simulink model "suspension"  (R2019a)
settings: Solver=ode15s  StartTime=0.0  StopTime=60  MaxStep=0.01  RelTol=1e-3  EnableMultiTasking=on
model workspace (MATLAB code in the model file):
  | dgrey = [0.3 0.3 0.3];
  | lgrey = [0.6 0.6 0.6];
  | orange = [255 140 0]/255;
  | blue = [0.0 0.6 0.8];
  | brown = [0.3 0.2 0.0];
  | lbrown = [167 108 52]/255;
  | yellow = [0.9 0.7 0.2];
  | red = [1.0 0.2 0.2];
  | black = [0 0 0];
  | 
  | rho_alum = 2700;
values from neighbouring files (symbols this model uses):
  back_frame_rad = intocm(0.25)    [loading.m]
  back_frame_thick_frame = intocm(0.25)    [loading.m]
  brake_disk_rad = intocm(3)    [loading.m]
  brake_disk_thick = intocm(0.25)    [loading.m]
  front_frame_rad = intocm(0.25)    [loading.m]
  front_frame_thick_frame = intocm(0.25)    [loading.m]
  hub_radius = intocm(2)    [loading.m]
  lower_left_link_len = intocm(link_upper)    [loading.m]
  lower_right_link_len = intocm(link_upper)    [loading.m]
  max_angle = 35    [loading.m]
  num_spokes = 4    [loading.m]
  outer_radius_spokes = intocm(5)    [loading.m]
  shaft_len = intocm(8)    [loading.m]
  shaft_rad = intocm(1.5)    [loading.m]
  steer_arm_chamfer = 0.25    [loading.m]
  steer_arm_height_forked = 13    [loading.m]
  steer_arm_len = 20    [loading.m]
  steer_arm_len_forked = 4    [loading.m]
  steer_arm_offset_forked = 3    [loading.m]
  steer_arm_pin_rad = 0.25    [loading.m]
  steer_arm_thick = 1    [loading.m]
  steer_arm_width = 2    [loading.m]
  steering_ball_rad = 1    [loading.m]
  steering_pin_height = 3    [loading.m]
  steering_pin_rad = 0.5    [loading.m]
  thickness_spokes = intocm(1)    [loading.m]
  tire_chamfer = 1    [loading.m]
  tire_density = 1000    [loading.m]
  tire_radius = intocm(9)    [loading.m]
  tire_width = intocm(7.5)    [loading.m]
  Ts = 60    [loading.m]
  upper_left_link_len = intocm(link_upper)    [loading.m]
  upper_right_link_len = intocm(link_upper)    [loading.m]
  upright_bearing_housing = 6    [loading.m]
  upright_chamfer = 0.3    [loading.m]
  upright_heigh_wheel = 8    [loading.m]
  upright_height = 43    [loading.m]
  upright_hub_thick = 2.5    [loading.m]
  upright_len = 8    [loading.m]
  upright_shaft_rad = 2.5    [loading.m]
  upright_thickness = 1    [loading.m]
  upright_trans_rad_to_wheel = 2    [loading.m]
  upright_width_wishbone = 10    [loading.m]
  width_hub = intocm(4.5)    [loading.m]
undefined symbols (not defined in the file or in its folder): sm_dwb_roadgen, X, Y, Z
libraries: sm_lib x75, sm_double_wishbone_suspension_lib x23, nesl_utility x18, simulink x3
(part 2 of 4)

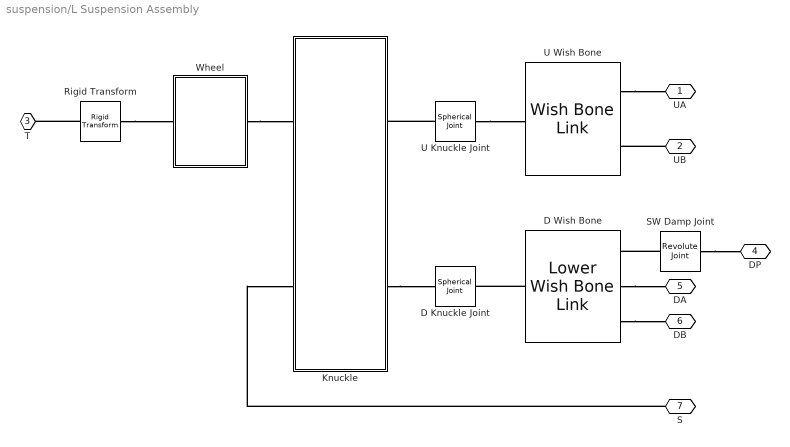
== system suspension/L Suspension Assembly ==
  D Knuckle Joint : sm_lib/Joints/Spherical Joint  SenseConstraintForce=off  SenseConstraintForceX=off  SenseConstraintForceY=off  SenseConstraintForceZ=off  SenseConstraintTorque=off  SenseConstraintTorqueX=off  SenseConstraintTorqueY=off  SenseConstraintTorqueZ=off  SenseTotalForce=off  SenseTotalForceX=off  SenseTotalForceY=off  SenseTotalForceZ=off  SenseTotalTorque=off  SenseTotalTorqueX=off  SenseTotalTorqueY=off  SenseTotalTorqueZ=off  CompositeWrenchDir=FollowerOnBase  CompositeWrenchFrame=BaseFrame  DefPosRotationMethod=None  DefPosRotationAngleUnits=deg  DefPosRotationStandardAxis=+Z  DefPosRotationAngle=0  DefPosRotationArbitraryAxis=[0 0 1]  DefPosFollAlignAxisA=+X  DefPosBaseAlignAxisA=+Y  DefPosFollAlignAxisB=+Y  DefPosBaseAlignAxisB=+Z  DefPosRotationSequenceAxes=FollowerAxes  DefPosRotationSequence=XYX  DefPosRotationSequenceAngles=[0 0 0]  DefPosRotationSequenceAnglesUnits=deg  DefPosRotationMatrix=[1 0 0; 0 1 0; 0 0 1]  EqPosRotationMethod=None  EqPosRotationAngleUnits=deg  EqPosRotationStandardAxis=+Z  EqPosRotationAngle=0  EqPosRotationArbitraryAxis=[0 0 1]  EqPosFollAlignAxisA=+X  EqPosBaseAlignAxisA=+Y  EqPosFollAlignAxisB=+Y  EqPosBaseAlignAxisB=+Z  EqPosRotationSequenceAxes=FollowerAxes  EqPosRotationSequence=XYX  EqPosRotationSequenceAngles=[0 0 0]  EqPosRotationSequenceAnglesUnits=deg  EqPosRotationMatrix=[1 0 0; 0 1 0; 0 0 1]  SpringStiffness=0  SpringStiffnessUnits=N*m/deg  DampingCoefficient=0  DampingCoefficientUnits=N*m/(deg/s)  ActuateTorqueX=off  ActuateTorqueY=off  ActuateTorqueZ=off  ActuateTorque=off  TorqueActuationMode=NoTorque  MotionActuationMode=ComputedMotion  ActuationFrame=BaseFrame  SensePosition=off  SenseVelocityX=off  SenseVelocityY=off  SenseVelocityZ=off  SenseVelocity=off  SenseAccelerationX=off  SenseAccelerationY=off  SenseAccelerationZ=off  SenseAcceleration=off  SenseTorqueX=off  SenseTorqueY=off  SenseTorqueZ=off  SenseTorqueForce=off  SenseLowerLimitTorqueMag=off  SenseUpperLimitTorqueMag=off  SensingFrame=BaseFrame  LowerLimitSpecify=off  LowerLimitBound=15  LowerLimitBoundUnits=deg  LowerLimitStiffness=1e4  LowerLimitStiffnessUnits=N*m/deg  LowerLimitDamping=10  LowerLimitDampingUnits=N*m/(deg/s)  LowerLimitTransitionRegionWidth=0.1  LowerLimitTransitionRegionWidthUnits=deg  UpperLimitSpecify=off  UpperLimitBound=45  UpperLimitBoundUnits=deg  UpperLimitStiffness=1e4  UpperLimitStiffnessUnits=N*m/deg  UpperLimitDamping=10  UpperLimitDampingUnits=N*m/(deg/s)  UpperLimitTransitionRegionWidth=0.1  UpperLimitTransitionRegionWidthUnits=deg  PositionTargetRotationMethod=None  PositionTargetRotationAngleUnits=deg  PositionTargetRotationStandardAxis=+Z  PositionTargetRotationAngle=0  PositionTargetRotationArbitraryAxis=[0 0 1]  PositionTargetFollAlignAxisA=+Y  PositionTargetBaseAlignAxisA=-Y  PositionTargetFollAlignAxisB=+Z  PositionTargetBaseAlignAxisB=-Z  PositionTargetRotationSequenceAxes=FollowerAxes  PositionTargetRotationSequence=XYX  PositionTargetRotationSequenceAngles=[0 0 0]  PositionTargetRotationSequenceAnglesUnits=deg  PositionTargetRotationMatrix=[1 0 0; 0 1 0; 0 0 1]  PositionTargetSpecify=off  PositionTargetPriority=Low  VelocityTargetValue=[0 0 0]  VelocityTargetValueUnits=deg/s  VelocityTargetSpecify=off  VelocityTargetPriority=High  VelocityTargetInFollowerFrame=on
  D Wish Bone : sm_double_wishbone_suspension_lib/Lower Wish Bone Link  L1=36  L2=25  L3=5  W3=5  W=14.75  T=2  Rb=2.875  Ob=15  Rev=on  Lb=4  Rsh=0.75  Rs=2  Hi=1.4  Rh=1  Oh=3.0625  Odb=10  Wdb=4  Ldb=4  Tdb=1  Sdb=1.5  Rhdb=1  rho=rho_alum  clr=lbrown
      settings: SourceProductName=Simscape Multibody  SourceProductBaseCode=MS
  Knuckle : Subsystem  mask(Steering knuckle){H=upright_height, L=upright_len, T=upright_thickness, Wpr=upright_hub_thick, Hpr=upright_heigh_wheel, Wc=upright_width_wishbone, Rd=upright_shaft_rad, Hd=upright_bearing_housing, Rr=upright_chamfer, Rt=upright_trans_rad_to_wheel, Rb=steering_ball_rad, Rp=steering_pin_rad, Hp=steering_pin_height, Ls=steer_arm_len, Ws=steer_arm_width, Ts=steer_arm_thick, Hsf=steer_arm_height_forked, Lsf=steer_arm_len_forked, Osf=steer_arm_offset_forked, Rsp=steer_arm_pin_rad, Rsr=steer_arm_chamfer, Rev=on, rho=rho_alum, clr=dgrey}
      mask prompts: H "Height (cm):"; L "Length (cm):"; T "Thickness (cm):"; Wpr "Width of wheel attach projection (cm):"; Hpr "Height of wheel attach projection (cm):"; Wc "Width of wishbone connectors (cm):"; Rd "Drive shaft hole radius (cm):"; Hd "Drive shaft bearing housing height (cm):"; Rr "Chamfer/fillet radius (cm):"; Rt "Transition radius to wheel attach projection (cm):"; Rb "Ball radius (cm):"; Rp "Pin radius (cm):"; Hp "Pin height (cm):"; Ls "Length of arm (cm):"; Ws "Width of arm (cm):"; Ts "Thickness of arm (cm):"; Hsf "Height of forked section (cm):"; Lsf "Length of forked section (cm):"; Osf "Offset of forked section (cm):"; Rsp "Pin radius (cm):"; Rsr "Chamfer/fillet radius (cm):"; Rev "Reverse direction:"; rho "Density (kg/m^3):"; clr "Color [r g b]:"
      mask help: This block models a steering knuckle. The wheel hub attaches to the steering knuckle. The steering knuckle attaches to the wishbone links. The ports U and D correspond to the frames where the knucle connects to the wishbone links. The port W corresponds to the frame where the wheel hub attaches to the knuckle. The knuckle also has a rigidly attached steering arm that attaches to the steering rack via tie rods. The port S corresponds to the frame where the steering arm attaches to the tie rod.
      mask init:
      | s_knuckle_xsec = [0 -Hd/2; 0 -Hpr/2; Wpr -Hpr/2; Wpr -H/2;
      |                 Wpr+Wc -H/2; Wpr+Wc -H/2+T; Wpr+T -H/2+T;
      |                  Wpr+T -Hd/2];
      | 
      | s_knuckle_xsec = simmechanics.demohelpers.round_corners(s_knuckle_xsec, 2:7, ...
      |                              [Rr Rt Rr*ones(1,4)], 20);
      | 
      | n_knuckle_xsec = flipud([s_knuckle_xsec(:,1) -s_knuckle_xsec(:,2)]);                         
      | 
      | Roh = sqrt((L/2)^2 + (Hd/2)^2);
      | phi = atan2(Hd,L);
      | theta = linspace(pi/2-phi,pi/2+phi,50)';
      | sh_xsec = [Roh*cos(theta) Roh*sin(theta)];
      | theta = linspace(3*pi/2-phi,3*pi/2+phi,50)';
      | sh_xsec = [sh_xsec; Roh*cos(theta) Roh*sin(theta)];
      | theta = linspace(5*pi/2-phi,pi/2-phi,100)';
      | sh_xsec = [sh_xsec; sh_xsec(1,:); Rd*cos(theta) Rd*sin(theta)];
      | 
      | % Convert Rev variable into +/- 1 instead of 0 or 1
      | sgn = (2*Rev-1);
      mask Display:
      | image(imread('sm_dwishbone_knuckle.png'));
      | port_label('RConn',1,'U');
      | port_label('RConn',2,'D');
      | port_label('LConn',1,'W');
      | port_label('LConn',2,'S');
  Rigid Transform : sm_lib/Frames and Transforms/Rigid Transform  TranslationMethod=None  TranslationStandardOffset=0  TranslationLengthUnit=m  TranslationStandardAxis=+Z  TranslationCartesianOffset=[0 0 0]  TranslationROffset=0  TranslationROffsetUnits=m  TranslationZOffset=0  TranslationZOffsetUnits=m  TranslationThetaOffset=0  TranslationThetaOffsetUnits=deg  RotationMethod=AlignedAxes  RotationAngleUnits=deg  RotationStandardAxis=+Z  RotationAngle=0  RotationArbitraryAxis=[0 0 1]  FollAlignAxisA=+X  BaseAlignAxisA=-X  FollAlignAxisB=+Z  BaseAlignAxisB=+Z  RotationSequenceAxes=FollowerAxes  RotationSequence=XYX  RotationSequenceAngles=[0 0 0]  RotationSequenceAnglesUnits=deg  RotationMatrix=[1 0 0; 0 1 0; 0 0 1]
  SW Damp Joint : sm_lib/Joints/Revolute Joint  SenseConstraintForce=off  SenseConstraintForceX=off  SenseConstraintForceY=off  SenseConstraintForceZ=off  SenseConstraintTorque=off  SenseConstraintTorqueX=off  SenseConstraintTorqueY=off  SenseConstraintTorqueZ=off  SenseTotalForce=off  SenseTotalForceX=off  SenseTotalForceY=off  SenseTotalForceZ=off  SenseTotalTorque=off  SenseTotalTorqueX=off  SenseTotalTorqueY=off  SenseTotalTorqueZ=off  CompositeWrenchDir=FollowerOnBase  CompositeWrenchFrame=BaseFrame  EquilibriumPosition=0  EquilibriumPositionUnits=deg  SpringStiffness=0  SpringStiffnessUnits=N*m/deg  DampingCoefficient=0  DampingCoefficientUnits=N*m/(deg/s)  TorqueActuationMode=NoTorque  MotionActuationMode=ComputedMotion  SensePosition=off  SenseVelocity=off  SenseAcceleration=off  SenseTorqueForce=off  SenseLowerLimitTorqueForce=off  SenseUpperLimitTorqueForce=off  LowerLimitSpecify=off  LowerLimitBound=-90  LowerLimitBoundUnits=deg  LowerLimitStiffness=1e4  LowerLimitStiffnessUnits=N*m/deg  LowerLimitDamping=10  LowerLimitDampingUnits=N*m/(deg/s)  LowerLimitTransitionRegionWidth=0.1  LowerLimitTransitionRegionWidthUnits=deg  UpperLimitSpecify=off  UpperLimitBound=90  UpperLimitBoundUnits=deg  UpperLimitStiffness=1e4  UpperLimitStiffnessUnits=N*m/deg  UpperLimitDamping=10  UpperLimitDampingUnits=N*m/(deg/s)  UpperLimitTransitionRegionWidth=0.1  UpperLimitTransitionRegionWidthUnits=deg  PositionTargetSpecify=on  PositionTargetPriority=Low  PositionTargetValue=-30  PositionTargetValueUnits=deg  VelocityTargetSpecify=off  VelocityTargetPriority=High  VelocityTargetValue=0  VelocityTargetValueUnits=deg/s
  U Knuckle Joint : sm_lib/Joints/Spherical Joint  SenseConstraintForce=off  SenseConstraintForceX=off  SenseConstraintForceY=off  SenseConstraintForceZ=off  SenseConstraintTorque=off  SenseConstraintTorqueX=off  SenseConstraintTorqueY=off  SenseConstraintTorqueZ=off  SenseTotalForce=off  SenseTotalForceX=off  SenseTotalForceY=off  SenseTotalForceZ=off  SenseTotalTorque=off  SenseTotalTorqueX=off  SenseTotalTorqueY=off  SenseTotalTorqueZ=off  CompositeWrenchDir=FollowerOnBase  CompositeWrenchFrame=BaseFrame  DefPosRotationMethod=None  DefPosRotationAngleUnits=deg  DefPosRotationStandardAxis=+Z  DefPosRotationAngle=0  DefPosRotationArbitraryAxis=[0 0 1]  DefPosFollAlignAxisA=+X  DefPosBaseAlignAxisA=+Y  DefPosFollAlignAxisB=+Y  DefPosBaseAlignAxisB=+Z  DefPosRotationSequenceAxes=FollowerAxes  DefPosRotationSequence=XYX  DefPosRotationSequenceAngles=[0 0 0]  DefPosRotationSequenceAnglesUnits=deg  DefPosRotationMatrix=[1 0 0; 0 1 0; 0 0 1]  EqPosRotationMethod=None  EqPosRotationAngleUnits=deg  EqPosRotationStandardAxis=+Z  EqPosRotationAngle=0  EqPosRotationArbitraryAxis=[0 0 1]  EqPosFollAlignAxisA=+X  EqPosBaseAlignAxisA=+Y  EqPosFollAlignAxisB=+Y  EqPosBaseAlignAxisB=+Z  EqPosRotationSequenceAxes=FollowerAxes  EqPosRotationSequence=XYX  EqPosRotationSequenceAngles=[0 0 0]  EqPosRotationSequenceAnglesUnits=deg  EqPosRotationMatrix=[1 0 0; 0 1 0; 0 0 1]  SpringStiffness=0  SpringStiffnessUnits=N*m/deg  DampingCoefficient=0  DampingCoefficientUnits=N*m/(deg/s)  ActuateTorqueX=off  ActuateTorqueY=off  ActuateTorqueZ=off  ActuateTorque=off  TorqueActuationMode=NoTorque  MotionActuationMode=ComputedMotion  ActuationFrame=BaseFrame  SensePosition=off  SenseVelocityX=off  SenseVelocityY=off  SenseVelocityZ=off  SenseVelocity=off  SenseAccelerationX=off  SenseAccelerationY=off  SenseAccelerationZ=off  SenseAcceleration=off  SenseTorqueX=off  SenseTorqueY=off  SenseTorqueZ=off  SenseTorqueForce=off  SenseLowerLimitTorqueMag=off  SenseUpperLimitTorqueMag=off  SensingFrame=BaseFrame  LowerLimitSpecify=off  LowerLimitBound=15  LowerLimitBoundUnits=deg  LowerLimitStiffness=1e4  LowerLimitStiffnessUnits=N*m/deg  LowerLimitDamping=10  LowerLimitDampingUnits=N*m/(deg/s)  LowerLimitTransitionRegionWidth=0.1  LowerLimitTransitionRegionWidthUnits=deg  UpperLimitSpecify=off  UpperLimitBound=45  UpperLimitBoundUnits=deg  UpperLimitStiffness=1e4  UpperLimitStiffnessUnits=N*m/deg  UpperLimitDamping=10  UpperLimitDampingUnits=N*m/(deg/s)  UpperLimitTransitionRegionWidth=0.1  UpperLimitTransitionRegionWidthUnits=deg  PositionTargetRotationMethod=AlignedAxes  PositionTargetRotationAngleUnits=deg  PositionTargetRotationStandardAxis=+Z  PositionTargetRotationAngle=0  PositionTargetRotationArbitraryAxis=[0 0 1]  PositionTargetFollAlignAxisA=+X  PositionTargetBaseAlignAxisA=-X  PositionTargetFollAlignAxisB=+Z  PositionTargetBaseAlignAxisB=-Z  PositionTargetRotationSequenceAxes=FollowerAxes  PositionTargetRotationSequence=XYX  PositionTargetRotationSequenceAngles=[0 0 0]  PositionTargetRotationSequenceAnglesUnits=deg  PositionTargetRotationMatrix=[1 0 0; 0 1 0; 0 0 1]  PositionTargetSpecify=off  PositionTargetPriority=High  VelocityTargetValue=[0 0 0]  VelocityTargetValueUnits=deg/s  VelocityTargetSpecify=off  VelocityTargetPriority=High  VelocityTargetInFollowerFrame=on
  U Wish Bone : sm_double_wishbone_suspension_lib/Wish Bone Link  L1=25  L2=15  L3=5  W3=5  W=25  T=2  Rb=8  Ob=5  Rev=on  Lb=4  Rsh=0.75  Rs=2  Hi=1.4  Rh=1  Oh=3  rho=rho_alum  clr=brown
      settings: SourceProductName=Simscape Multibody  SourceProductBaseCode=MS
  Wheel : Subsystem  mask(Wheel){Rti=outer_radius_spokes, Rto=tire_radius, Wt=tire_width, Rtr=tire_chamfer, trho=tire_density, tclr=black, Rhi=hub_radius, Rho=outer_radius_spokes, Ns=num_spokes, Ts=thickness_spokes, Wh=width_hub, Ls=shaft_len, Rs=shaft_rad, Rb=brake_disk_rad, Tb=brake_disk_thick, srho=rho_alum, sclr=yellow}
      mask prompts: Rti "Tire inner radius (cm):"; Rto "Tire outer radius (cm):"; Wt "Tire width (cm):"; Rtr "Chamfer/fillet radius (cm):"; trho "Density (kg/m^3):"; tclr "Color [r  g b]:"; Rhi "Hub radius (cm):"; Rho "Outer radius of spokes (cm):"; Ns "Number of spokes:"; Ts "Thickness of spokes:"; Wh "Width of hub (cm):"; Ls "Shaft length (cm):"; Rs "Shaft radius (cm):"; Rb "Brake disc radius (cm):"; Tb "Brake disc thickness (cm):"; srho "Density (kg/m^3):"; sclr "Color [r g b]:"
      mask help: This block models a wheel assembly. The port H corresponds to the center of the wheel hub.
      mask init:
      | spk_angles = linspace(0,2*pi,Ns+1);
      | 
      | spokes_xsec = [];
      | r_indices = [];
      | wang = 20*pi/180;
      | for idx = 1:length(spk_angles)-1
      |     ang = spk_angles(idx);
      |     theta = linspace(ang-wang,ang+wang,20)';
      |     spokes_xsec = [spokes_xsec;
      |                    Rhi*cos(theta) Rhi*sin(theta)];
      |     theta = linspace(ang+wang, spk_angles(idx+1)-wang, 50)';
      |     len = length(spokes_xsec);
      |     r_indices = [r_indices len len+1];
      |     spokes_xsec = [spokes_xsec;
      |                    Rho*cos(theta) Rho*sin(theta)];
      | end
      | 
      | rim_xsec = [Rho -Wh/2; Rti -Wt/2; 
      |             Rti Wt/2; Rho Wh/2+Ts];
      | 
      | tire_xsec = [Rti -Wt/2; Rto -Wt/2; Rto Wt/2; Rti Wt/2];
      | tire_xsec = simmechanics.demohelpers.round_corners(tire_xsec,1:4,Rtr,10);
      mask Display:
      | image(imread('sm_dwishbone_wheel.png'));
      | port_label('LConn',1,'H');
      | port_label('RConn',1,'T');
  UA : PMIOPort  Side=Right
  UB : PMIOPort  Port=2  Side=Right
  T : PMIOPort  Port=3  Side=Left
  DP : PMIOPort  Port=4  Side=Right
  DA : PMIOPort  Port=5  Side=Right
  DB : PMIOPort  Port=6  Side=Right
  S : PMIOPort  Port=7  Side=Right
  connections:
  D Wish Bone/RConn1 -- D Knuckle Joint/LConn1
  Wheel/LConn1 -- Knuckle/LConn1
  D Wish Bone/LConn3 -- DB/RConn1
  D Wish Bone/LConn2 -- DA/RConn1
  U Wish Bone/LConn1 -- UA/RConn1
  UB/RConn1 -- U Wish Bone/LConn2
  U Knuckle Joint/RConn1 -- Knuckle/RConn1
  U Knuckle Joint/LConn1 -- U Wish Bone/RConn1
  Rigid Transform/LConn1 -- Wheel/RConn1
  Rigid Transform/RConn1 -- T/RConn1
  S/RConn1 -- Knuckle/LConn2
  Knuckle/RConn2 -- D Knuckle Joint/RConn1
  SW Damp Joint/LConn1 -- D Wish Bone/LConn1
  SW Damp Joint/RConn1 -- DP/RConn1

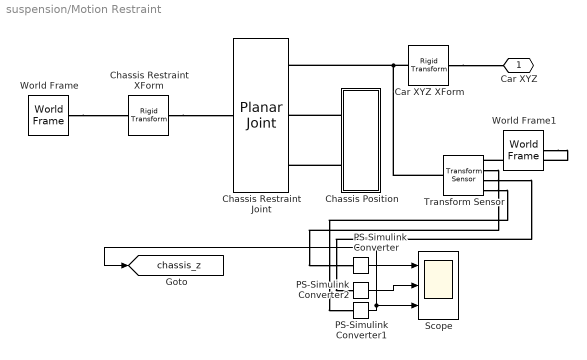
== system suspension/Motion Restraint ==
  Car XYZ XForm : sm_lib/Frames and Transforms/Rigid Transform  TranslationMethod=None  TranslationStandardOffset=0  TranslationLengthUnit=m  TranslationStandardAxis=+Z  TranslationCartesianOffset=[0 0 0]  TranslationROffset=0  TranslationROffsetUnits=m  TranslationZOffset=0  TranslationZOffsetUnits=m  TranslationThetaOffset=0  TranslationThetaOffsetUnits=deg  RotationMethod=AlignedAxes  RotationAngleUnits=deg  RotationStandardAxis=+Z  RotationAngle=0  RotationArbitraryAxis=[0 0 1]  FollAlignAxisA=+Y  BaseAlignAxisA=+X  FollAlignAxisB=+X  BaseAlignAxisB=+Z  RotationSequenceAxes=FollowerAxes  RotationSequence=XYX  RotationSequenceAngles=[0 0 0]  RotationSequenceAnglesUnits=deg  RotationMatrix=[1 0 0; 0 1 0; 0 0 1]
  Chassis Position : Subsystem
  Chassis Restraint XForm : sm_lib/Frames and Transforms/Rigid Transform  TranslationMethod=None  TranslationStandardOffset=0  TranslationLengthUnit=m  TranslationStandardAxis=+Z  TranslationCartesianOffset=[0 0 0]  TranslationROffset=0  TranslationROffsetUnits=m  TranslationZOffset=0  TranslationZOffsetUnits=m  TranslationThetaOffset=0  TranslationThetaOffsetUnits=deg  RotationMethod=AlignedAxes  RotationAngleUnits=deg  RotationStandardAxis=+Z  RotationAngle=0  RotationArbitraryAxis=[0 0 1]  FollAlignAxisA=+Y  BaseAlignAxisA=+Z  FollAlignAxisB=+X  BaseAlignAxisB=+X  RotationSequenceAxes=FollowerAxes  RotationSequence=XYX  RotationSequenceAngles=[0 0 0]  RotationSequenceAnglesUnits=deg  RotationMatrix=[1 0 0; 0 1 0; 0 0 1]
  Chassis Restraint Joint : sm_lib/Joints/Planar Joint  SenseConstraintForce=off  SenseConstraintForceX=off  SenseConstraintForceY=off  SenseConstraintForceZ=off  SenseConstraintTorque=off  SenseConstraintTorqueX=off  SenseConstraintTorqueY=off  SenseConstraintTorqueZ=off  SenseTotalForce=off  SenseTotalForceX=off  SenseTotalForceY=off  SenseTotalForceZ=off  SenseTotalTorque=off  SenseTotalTorqueX=off  SenseTotalTorqueY=off  SenseTotalTorqueZ=off  CompositeWrenchDir=FollowerOnBase  CompositeWrenchFrame=BaseFrame  PxEquilibriumPosition=0  PxEquilibriumPositionUnits=m  PxSpringStiffness=0  PxSpringStiffnessUnits=N/m  PxDampingCoefficient=0  PxDampingCoefficientUnits=N/(m/s)  PxTorqueActuationMode=NoTorque  PxMotionActuationMode=ComputedMotion  PxSensePosition=off  PxSenseVelocity=off  PxSenseAcceleration=off  PxSenseTorqueForce=off  PxSenseLowerLimitTorqueForce=off  PxSenseUpperLimitTorqueForce=off  PxLowerLimitSpecify=off  PxLowerLimitBound=-1  PxLowerLimitBoundUnits=m  PxLowerLimitStiffness=1e6  PxLowerLimitStiffnessUnits=N/m  PxLowerLimitDamping=1e3  PxLowerLimitDampingUnits=N/(m/s)  PxLowerLimitTransitionRegionWidth=1e-4  PxLowerLimitTransitionRegionWidthUnits=m  PxUpperLimitSpecify=off  PxUpperLimitBound=1  PxUpperLimitBoundUnits=m  PxUpperLimitStiffness=1e6  PxUpperLimitStiffnessUnits=N/m  PxUpperLimitDamping=1e3  PxUpperLimitDampingUnits=N/(m/s)  PxUpperLimitTransitionRegionWidth=1e-4  PxUpperLimitTransitionRegionWidthUnits=m  PxPositionTargetSpecify=off  PxPositionTargetPriority=High  PxPositionTargetValue=0  PxPositionTargetValueUnits=m  PxVelocityTargetSpecify=off  PxVelocityTargetPriority=High  PxVelocityTargetValue=0  PxVelocityTargetValueUnits=m/s  PyEquilibriumPosition=0  PyEquilibriumPositionUnits=m  PySpringStiffness=0  PySpringStiffnessUnits=N/m  PyDampingCoefficient=0  PyDampingCoefficientUnits=N/(m/s)  PyTorqueActuationMode=NoTorque  PyMotionActuationMode=ComputedMotion  PySensePosition=on  PySenseVelocity=off  PySenseAcceleration=off  PySenseTorqueForce=off  PySenseLowerLimitTorqueForce=off  PySenseUpperLimitTorqueForce=off  PyLowerLimitSpecify=off  PyLowerLimitBound=-1  PyLowerLimitBoundUnits=m  PyLowerLimitStiffness=1e6  PyLowerLimitStiffnessUnits=N/m  PyLowerLimitDamping=1e3  PyLowerLimitDampingUnits=N/(m/s)  PyLowerLimitTransitionRegionWidth=1e-4  PyLowerLimitTransitionRegionWidthUnits=m  PyUpperLimitSpecify=off  PyUpperLimitBound=1  PyUpperLimitBoundUnits=m  PyUpperLimitStiffness=1e6  PyUpperLimitStiffnessUnits=N/m  PyUpperLimitDamping=1e3  PyUpperLimitDampingUnits=N/(m/s)  PyUpperLimitTransitionRegionWidth=1e-4  PyUpperLimitTransitionRegionWidthUnits=m  PyPositionTargetSpecify=on  PyPositionTargetPriority=High  PyPositionTargetValue=95  PyPositionTargetValueUnits=cm  PyVelocityTargetSpecify=off  PyVelocityTargetPriority=High  PyVelocityTargetValue=0  PyVelocityTargetValueUnits=m/s  RzEquilibriumPosition=0  RzEquilibriumPositionUnits=deg  RzSpringStiffness=0  RzSpringStiffnessUnits=N*m/deg  RzDampingCoefficient=0  RzDampingCoefficientUnits=N*m/(deg/s)  RzTorqueActuationMode=NoTorque  RzMotionActuationMode=ComputedMotion  RzSensePosition=on  RzSenseVelocity=off  RzSenseAcceleration=off  RzSenseTorqueForce=off  RzSenseLowerLimitTorqueForce=off  RzSenseUpperLimitTorqueForce=off  RzLowerLimitSpecify=off  RzLowerLimitBound=-90  RzLowerLimitBoundUnits=deg  RzLowerLimitStiffness=1e4  RzLowerLimitStiffnessUnits=N*m/deg  RzLowerLimitDamping=10  RzLowerLimitDampingUnits=N*m/(deg/s)  RzLowerLimitTransitionRegionWidth=0.1  RzLowerLimitTransitionRegionWidthUnits=deg  RzUpperLimitSpecify=off  RzUpperLimitBound=90  RzUpperLimitBoundUnits=deg  RzUpperLimitStiffness=1e4  RzUpperLimitStiffnessUnits=N*m/deg  RzUpperLimitDamping=10  RzUpperLimitDampingUnits=N*m/(deg/s)  RzUpperLimitTransitionRegionWidth=0.1  RzUpperLimitTransitionRegionWidthUnits=deg  RzPositionTargetSpecify=on  RzPositionTargetPriority=High  RzPositionTargetValue=0  RzPositionTargetValueUnits=deg  RzVelocityTargetSpecify=off  RzVelocityTargetPriority=High  RzVelocityTargetValue=0  RzVelocityTargetValueUnits=deg/s
  PS-Simulink Converter : nesl_utility/PS-Simulink Converter  PhysicalDomain=network_engine_domain  SubClassName=ps_output  LeftPortType=input  RightPortType=output  PseudoPeriodic=off  Frequencies=[]  Unit=m  AffineConversion=off
  PS-Simulink Converter1 : nesl_utility/PS-Simulink Converter  PhysicalDomain=network_engine_domain  SubClassName=ps_output  LeftPortType=input  RightPortType=output  PseudoPeriodic=off  Frequencies=[]  Unit=m  AffineConversion=off
  PS-Simulink Converter2 : nesl_utility/PS-Simulink Converter  PhysicalDomain=network_engine_domain  SubClassName=ps_output  LeftPortType=input  RightPortType=output  PseudoPeriodic=off  Frequencies=[]  Unit=1  AffineConversion=off
  Scope : Scope  NumInputPorts=3
  Transform Sensor : sm_lib/Frames and Transforms/Transform Sensor  MeasurementFrame=World  SenseAngle=off  SenseAxis=off  SenseAngle1=off  SenseAngle2=off  SenseAngle3=off  SenseQ=off  SenseR=off  SenseOmegaX=off  SenseOmegaY=off  SenseOmegaZ=off  SenseOmega1=off  SenseOmega2=off  SenseOmega3=off  SenseQDot=off  SenseRDot=off  SenseAlphaX=off  SenseAlphaY=off  SenseAlphaZ=off  SenseAlpha1=off  SenseAlpha2=off  SenseAlpha3=off  SenseQDDot=off  SenseRDDot=off  SenseX=on  SenseY=on  SenseZ=on  SenseRad=off  SenseAzim=off  SenseDist=off  SenseInc=off  SenseXDot=off  SenseYDot=off  SenseZDot=off  SenseRadDot=off  SenseAzimDot=off  SenseDistDot=off  SenseIncDot=off  SenseXDDot=off  SenseYDDot=off  SenseZDDot=off  SenseRadDDot=off  SenseAzimDDot=off  SenseDistDDot=off  SenseIncDDot=off
  World Frame : sm_lib/Frames and Transforms/World Frame
  World Frame1 : sm_lib/Frames and Transforms/World Frame
  Car XYZ : PMIOPort  Side=Right
  tag scope: chassis_z=global
  wires:
  PS-Simulink Converter/1 -> Scope/1
  PS-Simulink Converter2/1 -> Scope/2
  PS-Simulink Converter1/1 -> [chassis_z], Scope/3
  connections:
  Chassis Position/LConn2 -- Chassis Restraint Joint/RConn3
  Chassis Position/LConn1 -- Chassis Restraint Joint/RConn2
  World Frame/RConn1 -- Chassis Restraint XForm/LConn1
  Chassis Restraint XForm/RConn1 -- Chassis Restraint Joint/LConn1
  Car XYZ XForm/RConn1 -- Car XYZ/RConn1
  Car XYZ XForm/LConn1 -- Transform Sensor/LConn1 -- Chassis Restraint Joint/RConn1
  World Frame1/RConn1 -- Transform Sensor/RConn1
  Transform Sensor/RConn4 -- PS-Simulink Converter1/LConn1
  Transform Sensor/RConn3 -- PS-Simulink Converter2/LConn1
  Transform Sensor/RConn2 -- PS-Simulink Converter/LConn1

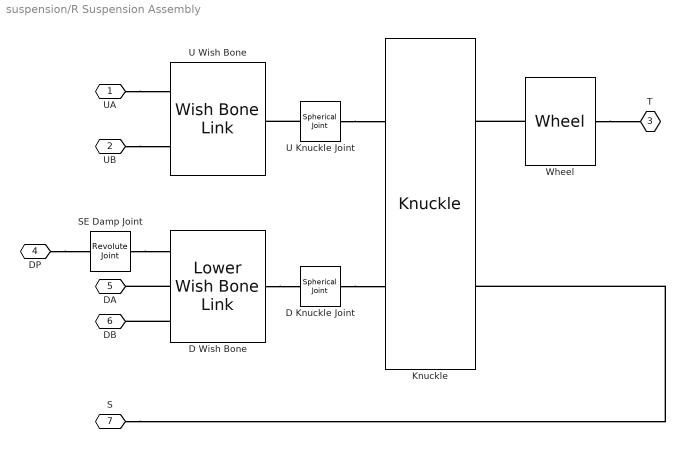
== system suspension/R Suspension Assembly ==
  D Knuckle Joint : sm_lib/Joints/Spherical Joint  SenseConstraintForce=off  SenseConstraintForceX=off  SenseConstraintForceY=off  SenseConstraintForceZ=off  SenseConstraintTorque=off  SenseConstraintTorqueX=off  SenseConstraintTorqueY=off  SenseConstraintTorqueZ=off  SenseTotalForce=off  SenseTotalForceX=off  SenseTotalForceY=off  SenseTotalForceZ=off  SenseTotalTorque=off  SenseTotalTorqueX=off  SenseTotalTorqueY=off  SenseTotalTorqueZ=off  CompositeWrenchDir=FollowerOnBase  CompositeWrenchFrame=BaseFrame  DefPosRotationMethod=None  DefPosRotationAngleUnits=deg  DefPosRotationStandardAxis=+Z  DefPosRotationAngle=0  DefPosRotationArbitraryAxis=[0 0 1]  DefPosFollAlignAxisA=+X  DefPosBaseAlignAxisA=+Y  DefPosFollAlignAxisB=+Y  DefPosBaseAlignAxisB=+Z  DefPosRotationSequenceAxes=FollowerAxes  DefPosRotationSequence=XYX  DefPosRotationSequenceAngles=[0 0 0]  DefPosRotationSequenceAnglesUnits=deg  DefPosRotationMatrix=[1 0 0; 0 1 0; 0 0 1]  EqPosRotationMethod=None  EqPosRotationAngleUnits=deg  EqPosRotationStandardAxis=+Z  EqPosRotationAngle=0  EqPosRotationArbitraryAxis=[0 0 1]  EqPosFollAlignAxisA=+X  EqPosBaseAlignAxisA=+Y  EqPosFollAlignAxisB=+Y  EqPosBaseAlignAxisB=+Z  EqPosRotationSequenceAxes=FollowerAxes  EqPosRotationSequence=XYX  EqPosRotationSequenceAngles=[0 0 0]  EqPosRotationSequenceAnglesUnits=deg  EqPosRotationMatrix=[1 0 0; 0 1 0; 0 0 1]  SpringStiffness=0  SpringStiffnessUnits=N*m/deg  DampingCoefficient=0  DampingCoefficientUnits=N*m/(deg/s)  ActuateTorqueX=off  ActuateTorqueY=off  ActuateTorqueZ=off  ActuateTorque=off  TorqueActuationMode=NoTorque  MotionActuationMode=ComputedMotion  ActuationFrame=BaseFrame  SensePosition=off  SenseVelocityX=off  SenseVelocityY=off  SenseVelocityZ=off  SenseVelocity=off  SenseAccelerationX=off  SenseAccelerationY=off  SenseAccelerationZ=off  SenseAcceleration=off  SenseTorqueX=off  SenseTorqueY=off  SenseTorqueZ=off  SenseTorqueForce=off  SenseLowerLimitTorqueMag=off  SenseUpperLimitTorqueMag=off  SensingFrame=BaseFrame  LowerLimitSpecify=off  LowerLimitBound=15  LowerLimitBoundUnits=deg  LowerLimitStiffness=1e4  LowerLimitStiffnessUnits=N*m/deg  LowerLimitDamping=10  LowerLimitDampingUnits=N*m/(deg/s)  LowerLimitTransitionRegionWidth=0.1  LowerLimitTransitionRegionWidthUnits=deg  UpperLimitSpecify=off  UpperLimitBound=45  UpperLimitBoundUnits=deg  UpperLimitStiffness=1e4  UpperLimitStiffnessUnits=N*m/deg  UpperLimitDamping=10  UpperLimitDampingUnits=N*m/(deg/s)  UpperLimitTransitionRegionWidth=0.1  UpperLimitTransitionRegionWidthUnits=deg  PositionTargetRotationMethod=None  PositionTargetRotationAngleUnits=deg  PositionTargetRotationStandardAxis=+Z  PositionTargetRotationAngle=0  PositionTargetRotationArbitraryAxis=[0 0 1]  PositionTargetFollAlignAxisA=+X  PositionTargetBaseAlignAxisA=-X  PositionTargetFollAlignAxisB=+Y  PositionTargetBaseAlignAxisB=-Y  PositionTargetRotationSequenceAxes=FollowerAxes  PositionTargetRotationSequence=XYX  PositionTargetRotationSequenceAngles=[0 0 0]  PositionTargetRotationSequenceAnglesUnits=deg  PositionTargetRotationMatrix=[1 0 0; 0 1 0; 0 0 1]  PositionTargetSpecify=off  PositionTargetPriority=Low  VelocityTargetValue=[0 0 0]  VelocityTargetValueUnits=deg/s  VelocityTargetSpecify=off  VelocityTargetPriority=High  VelocityTargetInFollowerFrame=on
  D Wish Bone : sm_double_wishbone_suspension_lib/Lower Wish Bone Link  L1=36  L2=25  L3=5  W3=5  W=14.75  T=2  Rb=2.875  Ob=15  Rev=off  Lb=4  Rsh=0.75  Rs=2  Hi=1.4  Rh=1  Oh=3.0625  Odb=10  Wdb=4  Ldb=4  Tdb=1  Sdb=1.5  Rhdb=1  rho=rho_alum  clr=lbrown
      settings: SourceProductName=Simscape Multibody  SourceProductBaseCode=MS
  Knuckle : sm_double_wishbone_suspension_lib/Knuckle  H=43  L=8  T=1  Wpr=2.5  Hpr=8  Wc=10  Rd=2.5  Hd=6  Rr=0.3  Rt=2  Rb=1  Rp=0.5  Hp=3  Ls=20  Ws=2  Ts=1  Hsf=13  Lsf=4  Osf=3  Rsp=0.25  Rsr=0.25  Rev=off  rho=rho_alum  clr=dgrey
      settings: SourceProductName=Simscape Multibody  SourceProductBaseCode=MS
  SE Damp Joint : sm_lib/Joints/Revolute Joint  SenseConstraintForce=off  SenseConstraintForceX=off  SenseConstraintForceY=off  SenseConstraintForceZ=off  SenseConstraintTorque=off  SenseConstraintTorqueX=off  SenseConstraintTorqueY=off  SenseConstraintTorqueZ=off  SenseTotalForce=off  SenseTotalForceX=off  SenseTotalForceY=off  SenseTotalForceZ=off  SenseTotalTorque=off  SenseTotalTorqueX=off  SenseTotalTorqueY=off  SenseTotalTorqueZ=off  CompositeWrenchDir=FollowerOnBase  CompositeWrenchFrame=BaseFrame  EquilibriumPosition=0  EquilibriumPositionUnits=deg  SpringStiffness=0  SpringStiffnessUnits=N*m/deg  DampingCoefficient=0  DampingCoefficientUnits=N*m/(deg/s)  TorqueActuationMode=NoTorque  MotionActuationMode=ComputedMotion  SensePosition=off  SenseVelocity=off  SenseAcceleration=off  SenseTorqueForce=off  SenseLowerLimitTorqueForce=off  SenseUpperLimitTorqueForce=off  LowerLimitSpecify=off  LowerLimitBound=-90  LowerLimitBoundUnits=deg  LowerLimitStiffness=1e4  LowerLimitStiffnessUnits=N*m/deg  LowerLimitDamping=10  LowerLimitDampingUnits=N*m/(deg/s)  LowerLimitTransitionRegionWidth=0.1  LowerLimitTransitionRegionWidthUnits=deg  UpperLimitSpecify=off  UpperLimitBound=90  UpperLimitBoundUnits=deg  UpperLimitStiffness=1e4  UpperLimitStiffnessUnits=N*m/deg  UpperLimitDamping=10  UpperLimitDampingUnits=N*m/(deg/s)  UpperLimitTransitionRegionWidth=0.1  UpperLimitTransitionRegionWidthUnits=deg  PositionTargetSpecify=on  PositionTargetPriority=Low  PositionTargetValue=150  PositionTargetValueUnits=deg  VelocityTargetSpecify=off  VelocityTargetPriority=High  VelocityTargetValue=0  VelocityTargetValueUnits=deg/s
  U Knuckle Joint : sm_lib/Joints/Spherical Joint  SenseConstraintForce=off  SenseConstraintForceX=off  SenseConstraintForceY=off  SenseConstraintForceZ=off  SenseConstraintTorque=off  SenseConstraintTorqueX=off  SenseConstraintTorqueY=off  SenseConstraintTorqueZ=off  SenseTotalForce=off  SenseTotalForceX=off  SenseTotalForceY=off  SenseTotalForceZ=off  SenseTotalTorque=off  SenseTotalTorqueX=off  SenseTotalTorqueY=off  SenseTotalTorqueZ=off  CompositeWrenchDir=FollowerOnBase  CompositeWrenchFrame=BaseFrame  DefPosRotationMethod=None  DefPosRotationAngleUnits=deg  DefPosRotationStandardAxis=+Z  DefPosRotationAngle=0  DefPosRotationArbitraryAxis=[0 0 1]  DefPosFollAlignAxisA=+X  DefPosBaseAlignAxisA=+Y  DefPosFollAlignAxisB=+Y  DefPosBaseAlignAxisB=+Z  DefPosRotationSequenceAxes=FollowerAxes  DefPosRotationSequence=XYX  DefPosRotationSequenceAngles=[0 0 0]  DefPosRotationSequenceAnglesUnits=deg  DefPosRotationMatrix=[1 0 0; 0 1 0; 0 0 1]  EqPosRotationMethod=None  EqPosRotationAngleUnits=deg  EqPosRotationStandardAxis=+Z  EqPosRotationAngle=0  EqPosRotationArbitraryAxis=[0 0 1]  EqPosFollAlignAxisA=+X  EqPosBaseAlignAxisA=+Y  EqPosFollAlignAxisB=+Y  EqPosBaseAlignAxisB=+Z  EqPosRotationSequenceAxes=FollowerAxes  EqPosRotationSequence=XYX  EqPosRotationSequenceAngles=[0 0 0]  EqPosRotationSequenceAnglesUnits=deg  EqPosRotationMatrix=[1 0 0; 0 1 0; 0 0 1]  SpringStiffness=0  SpringStiffnessUnits=N*m/deg  DampingCoefficient=0  DampingCoefficientUnits=N*m/(deg/s)  ActuateTorqueX=off  ActuateTorqueY=off  ActuateTorqueZ=off  ActuateTorque=off  TorqueActuationMode=NoTorque  MotionActuationMode=ComputedMotion  ActuationFrame=BaseFrame  SensePosition=off  SenseVelocityX=off  SenseVelocityY=off  SenseVelocityZ=off  SenseVelocity=off  SenseAccelerationX=off  SenseAccelerationY=off  SenseAccelerationZ=off  SenseAcceleration=off  SenseTorqueX=off  SenseTorqueY=off  SenseTorqueZ=off  SenseTorqueForce=off  SenseLowerLimitTorqueMag=off  SenseUpperLimitTorqueMag=off  SensingFrame=BaseFrame  LowerLimitSpecify=off  LowerLimitBound=15  LowerLimitBoundUnits=deg  LowerLimitStiffness=1e4  LowerLimitStiffnessUnits=N*m/deg  LowerLimitDamping=10  LowerLimitDampingUnits=N*m/(deg/s)  LowerLimitTransitionRegionWidth=0.1  LowerLimitTransitionRegionWidthUnits=deg  UpperLimitSpecify=off  UpperLimitBound=45  UpperLimitBoundUnits=deg  UpperLimitStiffness=1e4  UpperLimitStiffnessUnits=N*m/deg  UpperLimitDamping=10  UpperLimitDampingUnits=N*m/(deg/s)  UpperLimitTransitionRegionWidth=0.1  UpperLimitTransitionRegionWidthUnits=deg  PositionTargetRotationMethod=AlignedAxes  PositionTargetRotationAngleUnits=deg  PositionTargetRotationStandardAxis=+Z  PositionTargetRotationAngle=0  PositionTargetRotationArbitraryAxis=[0 0 1]  PositionTargetFollAlignAxisA=+X  PositionTargetBaseAlignAxisA=-X  PositionTargetFollAlignAxisB=+Y  PositionTargetBaseAlignAxisB=-Y  PositionTargetRotationSequenceAxes=FollowerAxes  PositionTargetRotationSequence=XYX  PositionTargetRotationSequenceAngles=[0 0 0]  PositionTargetRotationSequenceAnglesUnits=deg  PositionTargetRotationMatrix=[1 0 0; 0 1 0; 0 0 1]  PositionTargetSpecify=off  PositionTargetPriority=High  VelocityTargetValue=[0 0 0]  VelocityTargetValueUnits=deg/s  VelocityTargetSpecify=off  VelocityTargetPriority=High  VelocityTargetInFollowerFrame=on
  U Wish Bone : sm_double_wishbone_suspension_lib/Wish Bone Link  L1=25  L2=15  L3=5  W3=5  W=25  T=2  Rb=8  Ob=5  Rev=off  Lb=4  Rsh=0.75  Rs=2  Hi=1.4  Rh=1  Oh=3  rho=rho_alum  clr=brown
      settings: SourceProductName=Simscape Multibody  SourceProductBaseCode=MS
  Wheel : sm_double_wishbone_suspension_lib/Wheel  Rti=30  Rto=40  Wt=15  Rtr=1  trho=1000  tclr=black  Rhi=5  Rho=28  Ns=5  Ts=1  Wh=11  Ls=10  Rs=2  Rb=10  Tb=1  srho=rho_alum  sclr=yellow
      settings: SourceProductName=Simscape Multibody  SourceProductBaseCode=MS
  UA : PMIOPort  Side=Left
  UB : PMIOPort  Port=2  Side=Left
  T : PMIOPort  Port=3  Side=Right
  DP : PMIOPort  Port=4  Side=Left
  DA : PMIOPort  Port=5  Side=Left
  DB : PMIOPort  Port=6  Side=Left
  S : PMIOPort  Port=7  Side=Left
  connections:
  D Wish Bone/RConn1 -- D Knuckle Joint/LConn1
  Wheel/LConn1 -- Knuckle/LConn1
  D Wish Bone/LConn3 -- DB/RConn1
  D Wish Bone/LConn2 -- DA/RConn1
  UA/RConn1 -- U Wish Bone/LConn1
  D Knuckle Joint/RConn1 -- Knuckle/RConn2
  U Knuckle Joint/RConn1 -- Knuckle/RConn1
  Wheel/RConn1 -- T/RConn1
  UB/RConn1 -- U Wish Bone/LConn2
  U Knuckle Joint/LConn1 -- U Wish Bone/RConn1
  S/RConn1 -- Knuckle/LConn2
  DP/RConn1 -- SE Damp Joint/LConn1
  SE Damp Joint/RConn1 -- D Wish Bone/LConn1

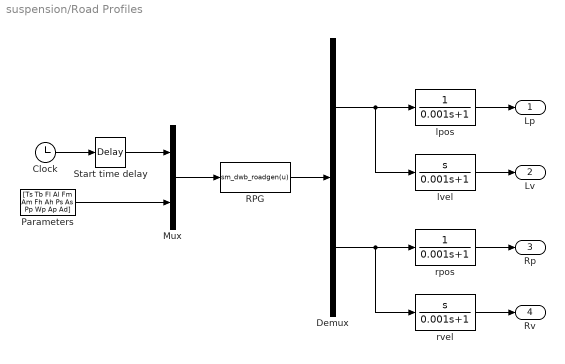
== system suspension/Road Profiles ==
  Clock : Clock
  Demux : Demux  Outputs=2
  Mux : Mux  Inputs=2
  Parameters : Constant  Value=[Ts Tb Fl Al Fm Am Fh Ah Ps As Pp Wp Ap Ad]
  RPG : MATLABFcn  MATLABFcn=sm_dwb_roadgen(u)
  Start time delay : TransportDelay  DelayTime=Ti
  lpos : TransferFcn  Denominator=[0.001 1]
  lvel : TransferFcn  Numerator=[1 0]  Denominator=[0.001 1]
  rpos : TransferFcn  Denominator=[0.001 1]
  rvel : TransferFcn  Numerator=[1 0]  Denominator=[0.001 1]
  Lp : Outport
  Lv : Outport  Port=2
  Rp : Outport  Port=3
  Rv : Outport  Port=4
  wires:
  Demux/1 -> lpos/1, lvel/1
  lpos/1 -> Lp/1
  lvel/1 -> Lv/1
  Demux/2 -> rvel/1, rpos/1
  rpos/1 -> Rp/1
  rvel/1 -> Rv/1
  Clock/1 -> Start time delay/1
  Parameters/1 -> Mux/2
  Mux/1 -> RPG/1
  RPG/1 -> Demux/1
  Start time delay/1 -> Mux/1

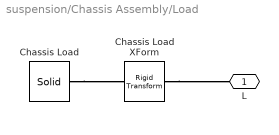
== system suspension/Chassis Assembly/Load ==
  Chassis Load : sm_lib/Body Elements/Solid  InertiaType=PointMass  Mass=600  MassUnits=kg  CenterOfMass=[0 0 0]  CenterOfMassUnits=m  MomentsOfInertia=[1 1 1]  MomentsOfInertiaUnits=kg*m^2  ProductsOfInertia=[0 0 0]  ProductsOfInertiaUnits=kg*m^2  BasedOnType=Mass  Density=1000  DensityUnits=kg/(m^3)  DoExposeReferenceFrame=on  SerializedFrames=<Frames/>  GraphicType=FromGeometry  MarkerShape=Sphere  MarkerSize=10  MarkerSizeUnits=m  GraphicVisPropType=SimpleVisualProperties  GraphicDiffuseColor=[0.6 0.0 0.0]  GraphicSpecularColor=[0.5 0.5 0.5 1.0]  GraphicAmbientColor=[0.15 0.15 0.15 1.0]  GraphicEmissiveColor=[0.0 0.0 0.0 1.0]  GraphicShininess=75  GraphicOpacity=1.0  GeometryShape=Brick  RectangleSize=[1 1]  RectangleSizeUnits=m  BrickDimensions=[5 5 5]  BrickDimensionUnits=cm  CylinderRadius=1  CylinderRadiusUnits=m  CylinderLength=1  CylinderLengthUnits=m  SphereRadius=1  SphereRadiusUnits=m  EllipsoidRadii=[1 1 1]  EllipsoidRadiiUnits=m  ExtrusionCrossSection=[1 1; -1 1; -1 -1; 1 -1]  ExtrusionCrossSectionUnits=m  ExtrusionLength=1  ExtrusionLengthUnits=m  PolygonNumSides=3  PolygonOuterRadius=1  PolygonOuterRadiusUnits=m  ExtGeomFileType=STL  ExtGeomFileUnits=m  RevolutionCrossSection=[1 1; 1 -1; 2 -1; 2 1]  RevolutionCrossSectionUnits=m  RevolutionExtent=Full  RevolutionAngle=180  RevolutionAngleUnits=deg
  Chassis Load XForm : sm_lib/Frames and Transforms/Rigid Transform  TranslationMethod=StandardAxis  TranslationStandardOffset=15  TranslationLengthUnit=cm  TranslationStandardAxis=+X  TranslationCartesianOffset=[0 0 0]  TranslationROffset=0  TranslationROffsetUnits=m  TranslationZOffset=0  TranslationZOffsetUnits=m  TranslationThetaOffset=0  TranslationThetaOffsetUnits=deg  RotationMethod=None  RotationAngleUnits=deg  RotationStandardAxis=+Z  RotationAngle=0  RotationArbitraryAxis=[0 0 1]  FollAlignAxisA=+X  BaseAlignAxisA=+Y  FollAlignAxisB=+Y  BaseAlignAxisB=+Z  RotationSequenceAxes=FollowerAxes  RotationSequence=XYX  RotationSequenceAngles=[0 0 0]  RotationSequenceAnglesUnits=deg  RotationMatrix=[1 0 0; 0 1 0; 0 0 1]
  L : PMIOPort  Side=Right
  connections:
  Chassis Load XForm/LConn1 -- L/RConn1
  Chassis Load/RConn1 -- Chassis Load XForm/RConn1

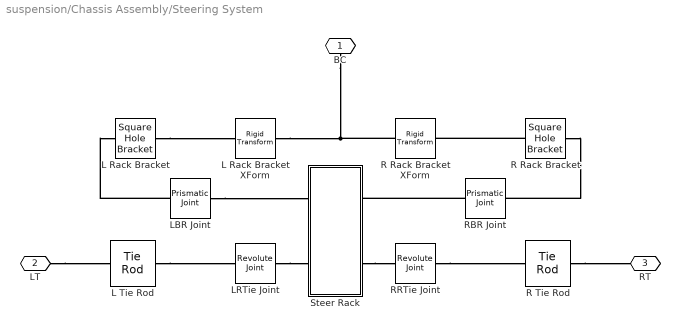
== system suspension/Chassis Assembly/Steering System ==
  L Rack Bracket : sm_double_wishbone_suspension_lib/Square Hole Bracket  L=4  W=4  T=4  Lh=2  Wh=2  Rr=0.5  rho=rho_alum  clr=orange
      settings: SourceProductName=Simscape Multibody  SourceProductBaseCode=MS
  L Rack Bracket XForm : sm_lib/Frames and Transforms/Rigid Transform  TranslationMethod=Cartesian  TranslationStandardOffset=0  TranslationLengthUnit=cm  TranslationStandardAxis=+X  TranslationCartesianOffset=[-1 -35 -18]  TranslationROffset=0  TranslationROffsetUnits=m  TranslationZOffset=0  TranslationZOffsetUnits=m  TranslationThetaOffset=0  TranslationThetaOffsetUnits=deg  RotationMethod=AlignedAxes  RotationAngleUnits=deg  RotationStandardAxis=+Z  RotationAngle=0  RotationArbitraryAxis=[0 0 1]  FollAlignAxisA=+Z  BaseAlignAxisA=-X  FollAlignAxisB=+X  BaseAlignAxisB=-Z  RotationSequenceAxes=FollowerAxes  RotationSequence=XYX  RotationSequenceAngles=[0 0 0]  RotationSequenceAnglesUnits=deg  RotationMatrix=[1 0 0; 0 1 0; 0 0 1]
  L Tie Rod : sm_double_wishbone_suspension_lib/Tie Rod  L=16.5  R=1.25  Rr=0.25  Lb=3  Wb=2  Tb=0.5  Sb=0.75  Rs=0.75  Rb=0.5  Rh=0.3  rho=rho_alum  tclr=yellow  bclr=brown
      settings: SourceProductName=Simscape Multibody  SourceProductBaseCode=MS
  LBR Joint : sm_lib/Joints/Prismatic Joint  SenseConstraintForce=off  SenseConstraintForceX=off  SenseConstraintForceY=off  SenseConstraintForceZ=off  SenseConstraintTorque=off  SenseConstraintTorqueX=off  SenseConstraintTorqueY=off  SenseConstraintTorqueZ=off  SenseTotalForce=off  SenseTotalForceX=off  SenseTotalForceY=off  SenseTotalForceZ=off  SenseTotalTorque=off  SenseTotalTorqueX=off  SenseTotalTorqueY=off  SenseTotalTorqueZ=off  CompositeWrenchDir=FollowerOnBase  CompositeWrenchFrame=BaseFrame  EquilibriumPosition=0  EquilibriumPositionUnits=m  SpringStiffness=10000  SpringStiffnessUnits=N/m  DampingCoefficient=500  DampingCoefficientUnits=N/(m/s)  TorqueActuationMode=NoTorque  MotionActuationMode=ComputedMotion  SensePosition=off  SenseVelocity=off  SenseAcceleration=off  SenseTorqueForce=off  SenseLowerLimitTorqueForce=off  SenseUpperLimitTorqueForce=off  LowerLimitSpecify=off  LowerLimitBound=-1  LowerLimitBoundUnits=m  LowerLimitStiffness=1e6  LowerLimitStiffnessUnits=N/m  LowerLimitDamping=1e3  LowerLimitDampingUnits=N/(m/s)  LowerLimitTransitionRegionWidth=1e-4  LowerLimitTransitionRegionWidthUnits=m  UpperLimitSpecify=off  UpperLimitBound=1  UpperLimitBoundUnits=m  UpperLimitStiffness=1e6  UpperLimitStiffnessUnits=N/m  UpperLimitDamping=1e3  UpperLimitDampingUnits=N/(m/s)  UpperLimitTransitionRegionWidth=1e-4  UpperLimitTransitionRegionWidthUnits=m  PositionTargetSpecify=off  PositionTargetPriority=High  PositionTargetValue=0  PositionTargetValueUnits=cm  VelocityTargetSpecify=off  VelocityTargetPriority=High  VelocityTargetValue=0  VelocityTargetValueUnits=m/s
  LRTie Joint : sm_lib/Joints/Revolute Joint  SenseConstraintForce=off  SenseConstraintForceX=off  SenseConstraintForceY=off  SenseConstraintForceZ=off  SenseConstraintTorque=off  SenseConstraintTorqueX=off  SenseConstraintTorqueY=off  SenseConstraintTorqueZ=off  SenseTotalForce=off  SenseTotalForceX=off  SenseTotalForceY=off  SenseTotalForceZ=off  SenseTotalTorque=off  SenseTotalTorqueX=off  SenseTotalTorqueY=off  SenseTotalTorqueZ=off  CompositeWrenchDir=FollowerOnBase  CompositeWrenchFrame=BaseFrame  EquilibriumPosition=0  EquilibriumPositionUnits=deg  SpringStiffness=0  SpringStiffnessUnits=N*m/deg  DampingCoefficient=0  DampingCoefficientUnits=N*m/(deg/s)  TorqueActuationMode=NoTorque  MotionActuationMode=ComputedMotion  SensePosition=off  SenseVelocity=off  SenseAcceleration=off  SenseTorqueForce=off  SenseLowerLimitTorqueForce=off  SenseUpperLimitTorqueForce=off  LowerLimitSpecify=off  LowerLimitBound=-90  LowerLimitBoundUnits=deg  LowerLimitStiffness=1e4  LowerLimitStiffnessUnits=N*m/deg  LowerLimitDamping=10  LowerLimitDampingUnits=N*m/(deg/s)  LowerLimitTransitionRegionWidth=0.1  LowerLimitTransitionRegionWidthUnits=deg  UpperLimitSpecify=off  UpperLimitBound=90  UpperLimitBoundUnits=deg  UpperLimitStiffness=1e4  UpperLimitStiffnessUnits=N*m/deg  UpperLimitDamping=10  UpperLimitDampingUnits=N*m/(deg/s)  UpperLimitTransitionRegionWidth=0.1  UpperLimitTransitionRegionWidthUnits=deg  PositionTargetSpecify=off  PositionTargetPriority=Low  PositionTargetValue=180  PositionTargetValueUnits=deg  VelocityTargetSpecify=off  VelocityTargetPriority=High  VelocityTargetValue=0  VelocityTargetValueUnits=deg/s
  R Rack Bracket : sm_double_wishbone_suspension_lib/Square Hole Bracket  L=4  W=4  T=4  Lh=2  Wh=2  Rr=0.5  rho=rho_alum  clr=orange
      settings: SourceProductName=Simscape Multibody  SourceProductBaseCode=MS
  R Rack Bracket XForm : sm_lib/Frames and Transforms/Rigid Transform  TranslationMethod=Cartesian  TranslationStandardOffset=0  TranslationLengthUnit=cm  TranslationStandardAxis=-X  TranslationCartesianOffset=[-1 35 -18]  TranslationROffset=0  TranslationROffsetUnits=m  TranslationZOffset=0  TranslationZOffsetUnits=m  TranslationThetaOffset=0  TranslationThetaOffsetUnits=deg  RotationMethod=AlignedAxes  RotationAngleUnits=deg  RotationStandardAxis=+Z  RotationAngle=0  RotationArbitraryAxis=[0 0 1]  FollAlignAxisA=+Z  BaseAlignAxisA=-X  FollAlignAxisB=+X  BaseAlignAxisB=-Z  RotationSequenceAxes=FollowerAxes  RotationSequence=XYX  RotationSequenceAngles=[0 0 0]  RotationSequenceAnglesUnits=deg  RotationMatrix=[1 0 0; 0 1 0; 0 0 1]
  R Tie Rod : sm_double_wishbone_suspension_lib/Tie Rod  L=16.5  R=1.25  Rr=0.25  Lb=3  Wb=2  Tb=0.5  Sb=0.75  Rs=0.75  Rb=0.5  Rh=0.3  rho=rho_alum  tclr=yellow  bclr=brown
      settings: SourceProductName=Simscape Multibody  SourceProductBaseCode=MS
  RBR Joint : sm_lib/Joints/Prismatic Joint  SenseConstraintForce=off  SenseConstraintForceX=off  SenseConstraintForceY=off  SenseConstraintForceZ=off  SenseConstraintTorque=off  SenseConstraintTorqueX=off  SenseConstraintTorqueY=off  SenseConstraintTorqueZ=off  SenseTotalForce=off  SenseTotalForceX=off  SenseTotalForceY=off  SenseTotalForceZ=off  SenseTotalTorque=off  SenseTotalTorqueX=off  SenseTotalTorqueY=off  SenseTotalTorqueZ=off  CompositeWrenchDir=FollowerOnBase  CompositeWrenchFrame=BaseFrame  EquilibriumPosition=0  EquilibriumPositionUnits=m  SpringStiffness=0  SpringStiffnessUnits=N/m  DampingCoefficient=0  DampingCoefficientUnits=N/(m/s)  TorqueActuationMode=NoTorque  MotionActuationMode=ComputedMotion  SensePosition=off  SenseVelocity=off  SenseAcceleration=off  SenseTorqueForce=off  SenseLowerLimitTorqueForce=off  SenseUpperLimitTorqueForce=off  LowerLimitSpecify=off  LowerLimitBound=-1  LowerLimitBoundUnits=m  LowerLimitStiffness=1e6  LowerLimitStiffnessUnits=N/m  LowerLimitDamping=1e3  LowerLimitDampingUnits=N/(m/s)  LowerLimitTransitionRegionWidth=1e-4  LowerLimitTransitionRegionWidthUnits=m  UpperLimitSpecify=off  UpperLimitBound=1  UpperLimitBoundUnits=m  UpperLimitStiffness=1e6  UpperLimitStiffnessUnits=N/m  UpperLimitDamping=1e3  UpperLimitDampingUnits=N/(m/s)  UpperLimitTransitionRegionWidth=1e-4  UpperLimitTransitionRegionWidthUnits=m  PositionTargetSpecify=off  PositionTargetPriority=High  PositionTargetValue=0  PositionTargetValueUnits=cm  VelocityTargetSpecify=off  VelocityTargetPriority=High  VelocityTargetValue=0  VelocityTargetValueUnits=m/s
  RRTie Joint : sm_lib/Joints/Revolute Joint  SenseConstraintForce=off  SenseConstraintForceX=off  SenseConstraintForceY=off  SenseConstraintForceZ=off  SenseConstraintTorque=off  SenseConstraintTorqueX=off  SenseConstraintTorqueY=off  SenseConstraintTorqueZ=off  SenseTotalForce=off  SenseTotalForceX=off  SenseTotalForceY=off  SenseTotalForceZ=off  SenseTotalTorque=off  SenseTotalTorqueX=off  SenseTotalTorqueY=off  SenseTotalTorqueZ=off  CompositeWrenchDir=FollowerOnBase  CompositeWrenchFrame=BaseFrame  EquilibriumPosition=0  EquilibriumPositionUnits=deg  SpringStiffness=0  SpringStiffnessUnits=N*m/deg  DampingCoefficient=0  DampingCoefficientUnits=N*m/(deg/s)  TorqueActuationMode=NoTorque  MotionActuationMode=ComputedMotion  SensePosition=off  SenseVelocity=off  SenseAcceleration=off  SenseTorqueForce=off  SenseLowerLimitTorqueForce=off  SenseUpperLimitTorqueForce=off  LowerLimitSpecify=off  LowerLimitBound=-90  LowerLimitBoundUnits=deg  LowerLimitStiffness=1e4  LowerLimitStiffnessUnits=N*m/deg  LowerLimitDamping=10  LowerLimitDampingUnits=N*m/(deg/s)  LowerLimitTransitionRegionWidth=0.1  LowerLimitTransitionRegionWidthUnits=deg  UpperLimitSpecify=off  UpperLimitBound=90  UpperLimitBoundUnits=deg  UpperLimitStiffness=1e4  UpperLimitStiffnessUnits=N*m/deg  UpperLimitDamping=10  UpperLimitDampingUnits=N*m/(deg/s)  UpperLimitTransitionRegionWidth=0.1  UpperLimitTransitionRegionWidthUnits=deg  PositionTargetSpecify=off  PositionTargetPriority=Low  PositionTargetValue=180  PositionTargetValueUnits=deg  VelocityTargetSpecify=off  VelocityTargetPriority=High  VelocityTargetValue=0  VelocityTargetValueUnits=deg/s
  Steer Rack : Subsystem  mask(Steering Rack){L=128, W=2, H=2, Db=70, Rr=0.5, Lb=4, Wb=2, Tb=0.5, Rh=0.5, rho=rho_alum, clr=brown}
      mask prompts: L "Length (cm):"; W "Width (cm):"; H "Height (cm):"; Db "Distance between holding brackets (cm):"; Rr "Chamfer/fillet radius (cm):"; Lb "Length (cm):"; Wb "Width (cm):"; Tb "Thickness (cm):"; Rh "Hole radius (cm):"; rho "Density (kg/m^3):"; clr "Color [r g b]:"
      mask help: This block models a steering rack with brackets at the end that connect to tie rods. The ports LT and RT correspond to the left and right tie rod frames. The ports LB and RB refer to the left and right holding bracket frames.
      mask init:
      | rack_xsec = [W/2 -H/2; W/2 H/2; -W/2 H/2; -W/2 -H/2];
      | rack_xsec = simmechanics.demohelpers.round_corners(rack_xsec,1:4,Rr,5);
      mask Display:
      | image(imread('sm_dwishbone_steerrack.png'));
      | port_label('LConn',1,'LB');
      | port_label('LConn',2,'LT');
      | port_label('RConn',1,'RB');
      | port_label('RConn',2,'RT');
  BC : PMIOPort  Side=Left
  LT : PMIOPort  Port=2  Side=Right
  RT : PMIOPort  Port=3  Side=Right
  connections:
  LBR Joint/RConn1 -- Steer Rack/LConn1
  R Rack Bracket/LConn1 -- R Rack Bracket XForm/RConn1
  Steer Rack/RConn2 -- RRTie Joint/LConn1
  R Rack Bracket/RConn1 -- RBR Joint/RConn1
  R Tie Rod/RConn1 -- RT/RConn1
  LRTie Joint/LConn1 -- Steer Rack/LConn2
  LBR Joint/LConn1 -- L Rack Bracket/RConn1
  L Tie Rod/LConn1 -- LRTie Joint/RConn1
  LT/RConn1 -- L Tie Rod/RConn1
  RRTie Joint/RConn1 -- R Tie Rod/LConn1
  RBR Joint/LConn1 -- Steer Rack/RConn1
  L Rack Bracket/LConn1 -- L Rack Bracket XForm/RConn1
  L Rack Bracket XForm/LConn1 -- BC/RConn1 -- R Rack Bracket XForm/LConn1
